simulink model "simple_delay_withoout_simulink_block"  (R2021a)
settings: Solver=VariableStepAuto  StartTime=0.0  StopTime=10.0  RelTol=1e-3
settings Model: Creator=DELL  LastModifiedBy=DELL

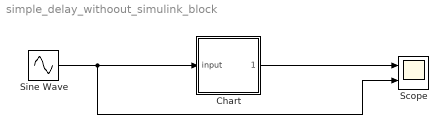
== system simple_delay_withoout_simulink_block ==
  Chart : Stateflow chart  TreatAsAtomicUnit=on
  Scope : Scope  NumInputPorts=2
  Sine Wave : Sin  SampleTime=0
  wires:
  Sine Wave/1 -> Chart/1(input), Scope/2
  Chart/1(output) -> Scope/1

== stateflow chart simple_delay_withoout_simulink_block/Chart ==
  (default) -> (junction 1) : {output=temp;temp=input;}
  data: output output double size=1; temp local double size=1; input input size=1
